simulink model "QuadRotor_Simulink"  (R2021a)
settings: Solver=ode23tb  StartTime=0.0  StopTime=1297.0156  RelTol=1e-3
undefined symbols (not defined in the file): QR_Object, QuadrotorBodyModel_Object, QuadrotorPowerTrainModel_Object
libraries: uavutilslib x1
settings Model: OrderedModelArguments=off  Creator=renkert2  LastModifiedBy=renkert2
settings SolverCC: AlgebraicLoopSolver=TrustRegion
settings DebuggingCC: SFMachineParentedDataDiag=warning

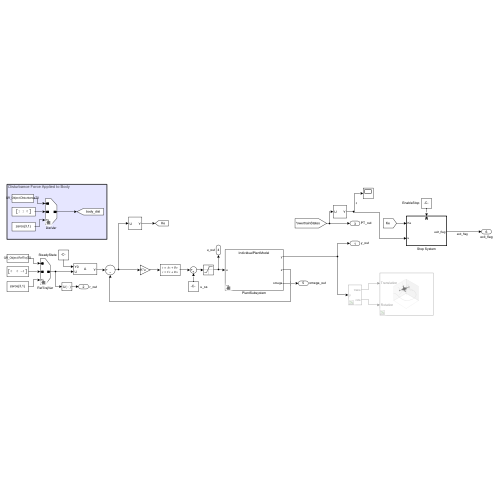
[thumbnail: Simulink's stored preview of the top-level diagram]
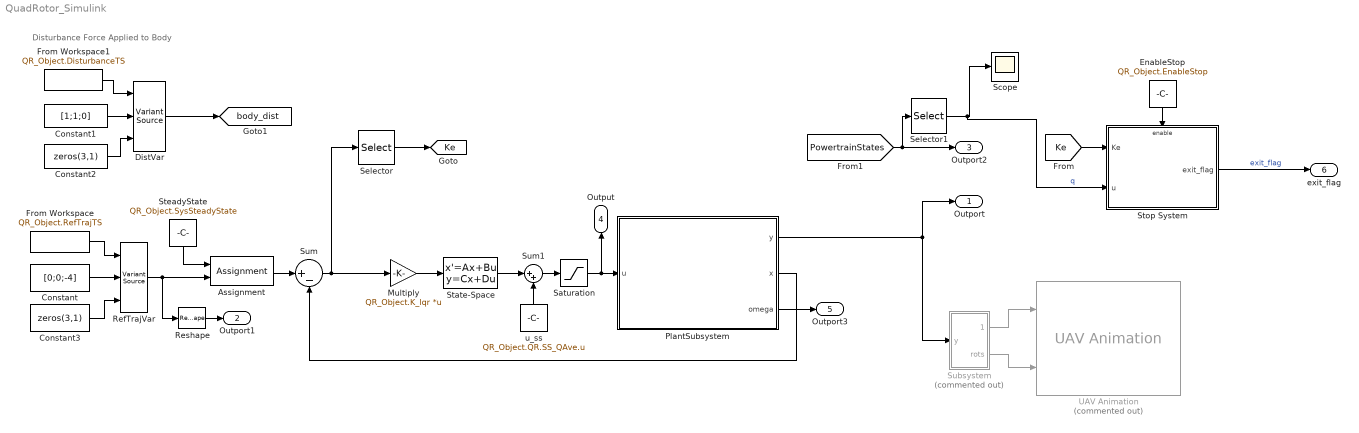
== system QuadRotor_Simulink ==
  note: Disturbance Force Applied to Body
  Assignment : Assignment  DiagnosticForDimensions=Warning  IndexOptions=Index vector (dialog)  Indices=5:7  OutputSizes=1
  Constant : Constant  Value=[0;0;-4]
  Constant1 : Constant  Value=[1;1;0]
  Constant2 : Constant  Value=zeros(3,1)
  Constant3 : Constant  Value=zeros(3,1)
  DistVar : VariantSource  VariantControlMode=label  LabelModeActiveChoice=Zeros
  EnableStop : Constant  Value=QR_Object.EnableStop  OutDataTypeStr=boolean
  From Workspace : FromWorkspace  VariableName=QR_Object.RefTrajTS  OutputAfterFinalValue=Holding final value
  From Workspace1 : FromWorkspace  VariableName=QR_Object.DisturbanceTS
  Multiply : Gain  Gain=QR_Object.K_lqr  Multiplication=Matrix(K*u)
  PlantSubsystem : Subsystem  Variant=on  VariantControlMode=label  LabelModeActiveChoice=Individual
  RefTrajVar : VariantSource  VariantControlMode=label  LabelModeActiveChoice=TimeSeries
  Reshape : Reshape
  Saturation : Saturate  UpperLimit=1  LowerLimit=0
  Scope : Scope
  Selector : Selector  InputPortWidth=16  IndexOptions=Index vector (dialog)  Indices=5:16  OutputSizes=1
  Selector1 : Selector  InputPortWidth=27  IndexOptions=Index vector (dialog)  Indices=1  OutputSizes=1
  State-Space : StateSpace  A=-1e6.*eye(4)  B=1e6.*eye(4)  C=eye(4)  D=zeros(4)  InitialCondition=0
  SteadyState : Constant  Value=QR_Object.SysSteadyState
  Stop System : Subsystem
  Subsystem : Subsystem  Commented=on
  Sum : Sum  Inputs=|+-
  Sum1 : Sum  Inputs=|++
  UAV Animation : uavutilslib/UAV Animation  Commented=on  UAVType=Multirotor  UAVSize=1  InertialZDirection=Down  SampleTime=-1
      settings: SourceProductBaseCode=UV
  u_ss : Constant  Value=QR_Object.QR.SS_QAve.u  VectorParams1D=off
  Outport : Outport  SignalName=y_out
  Outport1 : Outport  Port=2  SignalName=r_out
  Outport2 : Outport  Port=3  SignalName=PT_out
  Output : Outport  Port=4  SignalName=u_out
  Outport3 : Outport  Port=5  SignalName=omega_out
  exit_flag : Outport  Port=6
  tag scope: Ke=global, body_dist=global
  wires:
  From Workspace/1 -> RefTrajVar/1
  Reshape/1 -> Outport1/1
  PlantSubsystem/1(y) -> Subsystem/1(y), Outport/1
  Sum/1 -> Selector/1, Multiply/1
  Constant/1 -> RefTrajVar/2
  SteadyState/1 -> Assignment/1
  Assignment/1 -> Sum/1
  RefTrajVar/1 -> Assignment/2, Reshape/1
  PlantSubsystem/2(x) -> Sum/2
  Subsystem/1(trans) -> UAV Animation/1
  Subsystem/2(rots) -> UAV Animation/2
  [PowertrainStates] -> Selector1/1, Outport2/1
  u_ss/1 -> Sum1/2
  Sum1/1 -> Saturation/1
  Saturation/1 -> Output/1, PlantSubsystem/1(u)
  PlantSubsystem/3(omega) -> Outport3/1
  Multiply/1 -> State-Space/1
  State-Space/1 -> Sum1/1
  Selector/1 -> [Ke]
  Selector1/1 -> Stop System/2(u), Scope/1  "q"
  EnableStop/1 -> Stop System/Enable
  [Ke] -> Stop System/1(Ke)
  DistVar/1 -> [body_dist]
  Constant1/1 -> DistVar/2
  From Workspace1/1 -> DistVar/1
  Constant2/1 -> DistVar/3
  Constant3/1 -> RefTrajVar/3
  Stop System/1(exit_flag) -> exit_flag/1  "exit_flag"

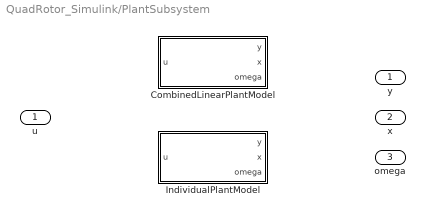
== system QuadRotor_Simulink/PlantSubsystem ==
  u : Inport
  CombinedLinearPlantModel : Subsystem  VariantControl=Combined
  IndividualPlantModel : Subsystem  VariantControl=Individual
  y : Outport
  x : Outport  Port=2
  omega : Outport  Port=3

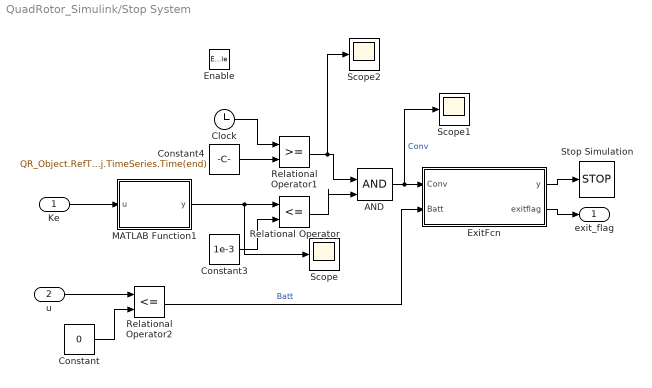
== system QuadRotor_Simulink/Stop System ==
  Ke : Inport
  u : Inport  Port=2
  Enable : EnablePort
  AND : Logic  IconShape=distinctive  AllPortsSameDT=off  OutDataTypeStr=boolean
  Clock : Clock
  Constant : Constant  Value=0
  Constant3 : Constant  Value=1e-3
  Constant4 : Constant  Value=QR_Object.RefTraj.TimeSeries.Time(end)
  ExitFcn : MATLAB Function  TreatAsAtomicUnit=on
  MATLAB Function1 : MATLAB Function  TreatAsAtomicUnit=on
  Relational Operator : RelationalOperator  Operator=<=  OutDataTypeStr=boolean  RndMeth=Simplest
  Relational Operator1 : RelationalOperator  OutDataTypeStr=boolean  RndMeth=Simplest
  Relational Operator2 : RelationalOperator  Operator=<=  OutDataTypeStr=boolean  RndMeth=Simplest
  Scope : Scope
  Scope1 : Scope
  Scope2 : Scope
  Stop Simulation : Stop
  exit_flag : Outport
  wires:
  Ke/1 -> MATLAB Function1/1(u)
  Constant4/1 -> Relational Operator1/2
  Relational Operator1/1 -> Scope2/1, AND/1
  MATLAB Function1/1(y) -> Scope/1, Relational Operator/1
  Clock/1 -> Relational Operator1/1
  Relational Operator/1 -> AND/2
  Constant3/1 -> Relational Operator/2
  ExitFcn/1(y) -> Stop Simulation/1
  u/1 -> Relational Operator2/1
  Constant/1 -> Relational Operator2/2
  Relational Operator2/1 -> ExitFcn/2(Batt)  "Batt"
  ExitFcn/2(exitflag) -> exit_flag/1
  AND/1 -> Scope1/1, ExitFcn/1(Conv)  "Conv"

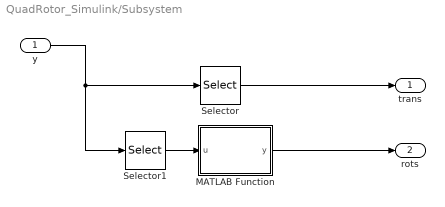
== system QuadRotor_Simulink/Subsystem ==
  y : Inport
  MATLAB Function : MATLAB Function  TreatAsAtomicUnit=on
  Selector : Selector  InputPortWidth=QuadrotorBodyModel_Object.Nx  IndexOptions=Index vector (dialog)  Indices=QuadrotorBodyModel_Object.I.x.p  OutputSizes=1
  Selector1 : Selector  InputPortWidth=QuadrotorBodyModel_Object.Nx  IndexOptions=Index vector (dialog)  Indices=QuadrotorBodyModel_Object.I.x.Theta  OutputSizes=1
  trans : Outport
  rots : Outport  Port=2
  wires:
  Selector/1 -> trans/1
  Selector1/1 -> MATLAB Function/1(u)
  y/1 -> Selector/1, Selector1/1
  MATLAB Function/1(y) -> rots/1

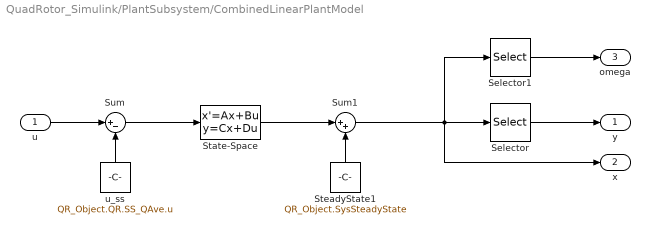
== system QuadRotor_Simulink/PlantSubsystem/CombinedLinearPlantModel ==
  u : Inport
  Selector : Selector  InputPortWidth=16  IndexOptions=Index vector (dialog)  Indices=5:16  OutputSizes=1
  Selector1 : Selector  InputPortWidth=16  IndexOptions=Index vector (dialog)  Indices=1:4  OutputSizes=1
  State-Space : StateSpace  A=QR_Object.LinearPlantModel.A  B=QR_Object.LinearPlantModel.B  C=QR_Object.LinearPlantModel.C  D=QR_Object.LinearPlantModel.D  InitialCondition=0
  SteadyState1 : Constant  Value=QR_Object.SysSteadyState
  Sum : Sum  Inputs=|+-
  Sum1 : Sum  Inputs=|++
  u_ss : Constant  Value=QR_Object.QR.SS_QAve.u  VectorParams1D=off
  y : Outport
  x : Outport  Port=2
  omega : Outport  Port=3
  wires:
  Sum1/1 -> Selector1/1, x/1, Selector/1
  Selector/1 -> y/1
  Selector1/1 -> omega/1
  u/1 -> Sum/1
  Sum/1 -> State-Space/1
  u_ss/1 -> Sum/2
  SteadyState1/1 -> Sum1/2
  State-Space/1 -> Sum1/1

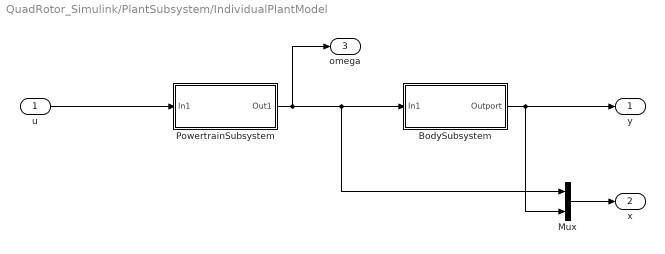
== system QuadRotor_Simulink/PlantSubsystem/IndividualPlantModel ==
  u : Inport
  BodySubsystem : Subsystem  Variant=on  VariantControlMode=label  LabelModeActiveChoice=Nonlinear
      settings: AttributesFormatString=%<CompiledVariantInfo>
  Mux : Mux  Inputs=2
  PowertrainSubsystem : Subsystem  Variant=on  VariantControlMode=label  LabelModeActiveChoice=Nonlinear
      settings: AttributesFormatString=%<CompiledVariantInfo>
  y : Outport
  x : Outport  Port=2
  omega : Outport  Port=3
  wires:
  PowertrainSubsystem/1(Out1) -> omega/1, BodySubsystem/1(In1), Mux/1
  u/1 -> PowertrainSubsystem/1(In1)
  Mux/1 -> x/1
  BodySubsystem/1(Outport) -> y/1, Mux/2

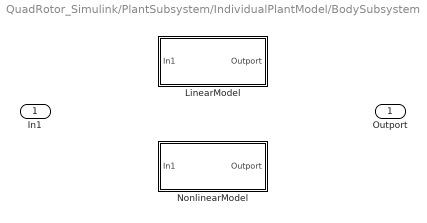
== system QuadRotor_Simulink/PlantSubsystem/IndividualPlantModel/BodySubsystem ==
  In1 : Inport
  LinearModel : Subsystem  VariantControl=Linear
  NonlinearModel : Subsystem  VariantControl=Nonlinear
  Outport : Outport

== system QuadRotor_Simulink/PlantSubsystem/IndividualPlantModel/PowertrainSubsystem ==
  In1 : Inport
  LinearModel : Subsystem  VariantControl=Linear
  NonlinearModel : Subsystem  VariantControl=Nonlinear
  Out1 : Outport

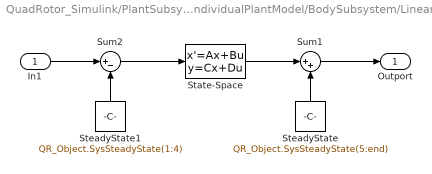
== system QuadRotor_Simulink/PlantSubsystem/IndividualPlantModel/BodySubsystem/LinearModel ==
  In1 : Inport
  State-Space : StateSpace  A=QR_Object.LinearBodyModel.A  B=QR_Object.LinearBodyModel.B  C=QR_Object.LinearBodyModel.C  D=QR_Object.LinearBodyModel.D  InitialCondition=0
  SteadyState : Constant  Value=QR_Object.SysSteadyState(5:end)
  SteadyState1 : Constant  Value=QR_Object.SysSteadyState(1:4)
  Sum1 : Sum  Inputs=|++
  Sum2 : Sum  Inputs=|+-
  Outport : Outport
  wires:
  State-Space/1 -> Sum1/1
  SteadyState/1 -> Sum1/2
  Sum1/1 -> Outport/1
  SteadyState1/1 -> Sum2/2
  In1/1 -> Sum2/1
  Sum2/1 -> State-Space/1

== system QuadRotor_Simulink/PlantSubsystem/IndividualPlantModel/BodySubsystem/NonlinearModel ==
  In1 : Inport
  QuadrotorBodyModel : Subsystem  mask{x_0=QuadrotorBodyModel_Object.x0}
  Outport : Outport
  wires:
  In1/1 -> QuadrotorBodyModel/1(Input1)
  QuadrotorBodyModel/1(Output) -> Outport/1
  [body_dist] -> QuadrotorBodyModel/2(Input2)

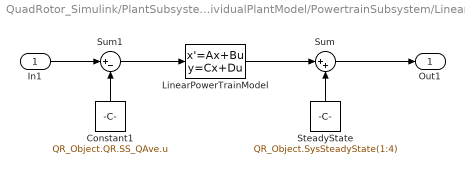
== system QuadRotor_Simulink/PlantSubsystem/IndividualPlantModel/PowertrainSubsystem/LinearModel ==
  In1 : Inport
  Constant1 : Constant  Value=QR_Object.QR.SS_QAve.u  VectorParams1D=off
  LinearPowerTrainModel : StateSpace  A=QR_Object.LinearPowertrainModel.A  B=QR_Object.LinearPowertrainModel.B  C=QR_Object.LinearPowertrainModel.C  D=QR_Object.LinearPowertrainModel.D  InitialCondition=0
  SteadyState : Constant  Value=QR_Object.SysSteadyState(1:4)
  Sum : Sum  Inputs=|++
  Sum1 : Sum  Inputs=|+-
  Out1 : Outport
  wires:
  LinearPowerTrainModel/1 -> Sum/1
  In1/1 -> Sum1/1
  Sum/1 -> Out1/1
  SteadyState/1 -> Sum/2
  Constant1/1 -> Sum1/2
  Sum1/1 -> LinearPowerTrainModel/1

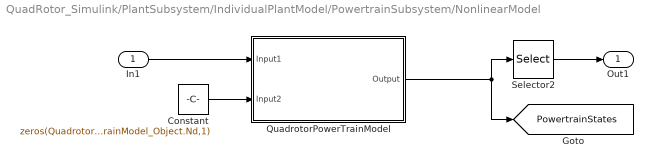
== system QuadRotor_Simulink/PlantSubsystem/IndividualPlantModel/PowertrainSubsystem/NonlinearModel ==
  In1 : Inport
  Constant : Constant  Value=zeros(QuadrotorPowerTrainModel_Object.Nd,1)
  QuadrotorPowerTrainModel : Subsystem  mask{x_0=QuadrotorPowerTrainModel_Object.x0}
  Selector2 : Selector  InputPortWidth=QuadrotorPowerTrainModel_Object.Ny  IndexOptions=Index vector (dialog)  Indices=QR_Object.QR.PT.SpeedOutputs_I  OutputSizes=1
  Out1 : Outport
  tag scope: PowertrainStates=global
  wires:
  QuadrotorPowerTrainModel/1(Output) -> [PowertrainStates], Selector2/1
  Selector2/1 -> Out1/1
  In1/1 -> QuadrotorPowerTrainModel/1(Input1)
  Constant/1 -> QuadrotorPowerTrainModel/2(Input2)

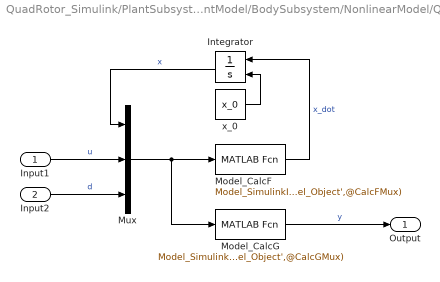
== system QuadRotor_Simulink/PlantSubsystem/IndividualPlantModel/BodySubsystem/NonlinearModel/QuadrotorBodyModel ==
  Input1 : Inport  PortDimensions=[QuadrotorBodyModel_Object.Nu,1]
  Input2 : Inport  Port=2  PortDimensions=[QuadrotorBodyModel_Object.Nd,1]
  Integrator : Integrator  InitialConditionSource=external
  Model_CalcF : MATLABFcn  MATLABFcn=Model_SimulinkInterpretedFunction(u,'QuadRotor_Simulink','QuadrotorBodyModel_Object',@CalcFMux)  OutputDimensions=QuadrotorBodyModel_Object.Nx
  Model_CalcG : MATLABFcn  MATLABFcn=Model_SimulinkInterpretedFunction(u,'QuadRotor_Simulink','QuadrotorBodyModel_Object',@CalcGMux)  OutputDimensions=QuadrotorBodyModel_Object.Ny
  Mux : Mux  Inputs=3
  x_0 : Constant  Value=x_0  VectorParams1D=off
  Output : Outport
  wires:
  Model_CalcF/1 -> Integrator/1  "x_dot"
  Input1/1 -> Mux/2  "u"
  Model_CalcG/1 -> Output/1  "y"
  x_0/1 -> Integrator/2
  Input2/1 -> Mux/3  "d"
  Integrator/1 -> Mux/1  "x"
  Mux/1 -> Model_CalcG/1, Model_CalcF/1

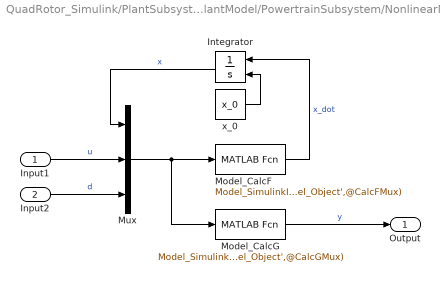
== system QuadRotor_Simulink/PlantSubsystem/IndividualPlantModel/PowertrainSubsystem/NonlinearModel/QuadrotorPowerTrainModel ==
  Input1 : Inport  PortDimensions=[QuadrotorPowerTrainModel_Object.Nu,1]
  Input2 : Inport  Port=2  PortDimensions=[QuadrotorPowerTrainModel_Object.Nd,1]
  Integrator : Integrator  InitialConditionSource=external
  Model_CalcF : MATLABFcn  MATLABFcn=Model_SimulinkInterpretedFunction(u,'QuadRotor_Simulink','QuadrotorPowerTrainModel_Object',@CalcFMux)  OutputDimensions=QuadrotorPowerTrainModel_Object.Nx
  Model_CalcG : MATLABFcn  MATLABFcn=Model_SimulinkInterpretedFunction(u,'QuadRotor_Simulink','QuadrotorPowerTrainModel_Object',@CalcGMux)  OutputDimensions=QuadrotorPowerTrainModel_Object.Ny
  Mux : Mux  Inputs=3
  x_0 : Constant  Value=x_0  VectorParams1D=off
  Output : Outport
  wires:
  Mux/1 -> Model_CalcF/1, Model_CalcG/1
  Integrator/1 -> Mux/1  "x"
  Input2/1 -> Mux/3  "d"
  x_0/1 -> Integrator/2
  Model_CalcG/1 -> Output/1  "y"
  Input1/1 -> Mux/2  "u"
  Model_CalcF/1 -> Integrator/1  "x_dot"

== matlab function QuadRotor_Simulink/Stop System/MATLAB Function1 ==
  data: u input; y output
function y = vecnorm(u)

y = norm(u,2)^2;
end

== matlab function QuadRotor_Simulink/Subsystem/MATLAB Function ==
  data: u input; y output
function y = eul2quatMF(u)
    y = eul2quat([1 -1 1].*fliplr(u'),'ZYX');
end

== matlab function QuadRotor_Simulink/Stop System/ExitFcn ==
  data: Conv input; y output; Batt input; exitflag output
function [y,exitflag] = ExitFcn(Conv,Batt)
y = false;
exitflag = 0;

if Conv
    % System converged to Steady-State
    disp("Simulation Converged: exitflag = 1")
    y = true;
    exitflag = 1; % System Converged
elseif Batt
    % Battery ran out
    disp("Simulation Stopped becuase Battery State-Of-Charge hit Lower Limit: exitflag = -1")
    y = true;
    exitflag = -1;
end
end
